simulink model "simSmc"  (R2015b)
settings: Solver=VariableStepAuto  StartTime=0.0  StopTime=10  RelTol=1e-3
InitFcn:
  | run smc.m
values from neighbouring files (symbols this model uses):
  A = [ 0 1; 0 -b]    [constants.m]    (also in smc.m = 500)
  a = g/l    (= 32.1639344262)    [constants.m]    (also in lyapRedesign.m = -10.9; smc.m = -32.1639344262)
  a1 = 12    [smc.m]
  a_hat = g/l_hat    (= -9.81)    [lyapRedesign.m]
  alpha = max(alpha_p)    [smc.m]
  b_hat = k_hat/m_hat    (= 0.151515151515)    [lyapRedesign.m]    (also in smc.m = mean(b_p))
  beta0 = ceil(Rho) - Rho    [smc.m]
  beta_wo_dis = beta_0_wo_dis + Rho_wo_dis    [smc.m]
  c_hat = 1/(m_hat*l_hat^2)    (= 1.51515151515)    [lyapRedesign.m]    (also in smc.m = mean(c_p))
  dt = 1/200    (= 0.005)    [smc.m]
  e = (xLimit/b)^2    (= 0.000625)    [lyapRedesign.m]    (also in smc.m = (x2_bound)/norm(1-1/theta))
  g = 9.81    [constants.m]    (also in lyapRedesign.m = -9.81; smc.m = -9.81)
  k1 = 40    [lyapRedesign.m]
  k2 = 40 - b_hat    (= 39.8484848485)    [lyapRedesign.m]
  Kf = min(Kf_p)    [smc.m]
  Km = 0.0934    [smc.m]
  l = 0.305    [constants.m]    (also in lyapRedesign.m = 0.9; smc.m)
  m = 0.1    [constants.m]    (also in lyapRedesign.m = 1.5; smc.m = min(m_p))
  rho1 = 1/c_hat * (abs((a_hat*c - a*c_hat)/c_hat) + abs((c*b_hat - c_hat*b)/c_hat) + k0*sqrt(5))    [lyapRedesign.m]    (also in smc.m = [abs( (1/c_hat - 1/max(c_p))*a ) abs( (a1-min(b_p))/min(c_p))
  rho2 = m_hat    (= 0.66)    [lyapRedesign.m]    (also in smc.m = (Km*A*(5/2000)/(min(m_p)*l))/min(c_p))
undefined symbols (not defined in the file or in its folder): DiscIntNeverNeededParam
settings Model: Creator=jn  LastModifiedBy=jn

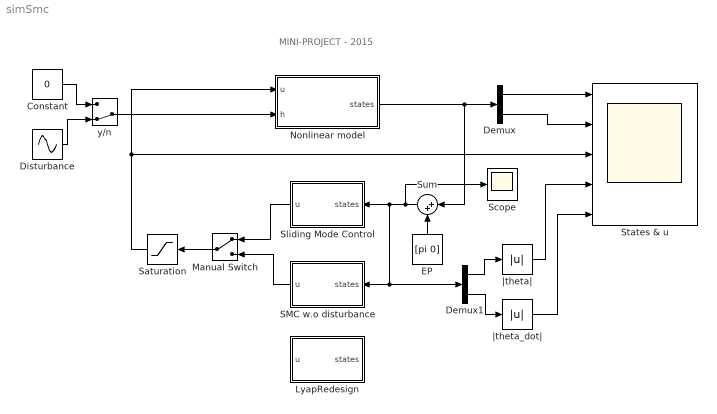
== system simSmc ==
  note: MINI-PROJECT - 2015
  Constant : Constant  Value=0
  Demux : Demux  Outputs=2
  Demux1 : Demux  Outputs=2
  Disturbance : Sin  Amplitude=Km*A*5/2000  SampleTime=0
  EP : Constant  Value=[pi 0]
  LyapRedesign : Subsystem
  Manual Switch : ManualSwitch
  Nonlinear model : Subsystem
  SMC w.o disturbance : Subsystem
  Saturation : Saturate  UpperLimit=2000  LowerLimit=-2000
  Scope : Scope
  Sliding Mode Control : Subsystem
  States & u : Scope  NumInputPorts=5
  Sum : Sum  Inputs=|++
  y/n : ManualSwitch  CurrentSetting=0
  |theta_dot| : Abs
  |theta| : Abs
  wires:
  Nonlinear model/1(states) -> Demux/1, Sum/1
  Demux/1 -> States & u/1
  Demux/2 -> States & u/2
  EP/1 -> Sum/2
  Sum/1 -> Scope/1, Sliding Mode Control/1(states), SMC w.o disturbance/1(states), Demux1/1
  Saturation/1 -> States & u/3, Nonlinear model/1(u)
  Demux1/1 -> |theta|/1
  Demux1/2 -> |theta_dot|/1
  |theta|/1 -> States & u/4
  |theta_dot|/1 -> States & u/5
  SMC w.o disturbance/1(u) -> Manual Switch/2
  Sliding Mode Control/1(u) -> Manual Switch/1
  Manual Switch/1 -> Saturation/1
  Disturbance/1 -> y/n/2
  Constant/1 -> y/n/1
  y/n/1 -> Nonlinear model/2(h)

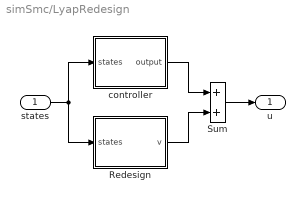
== system simSmc/LyapRedesign ==
  states : Inport
  Redesign : Subsystem
  Sum : Sum
  controller : Subsystem
  u : Outport
  wires:
  states/1 -> controller/1(states), Redesign/1(states)
  Redesign/1(v) -> Sum/2
  controller/1(output) -> Sum/1
  Sum/1 -> u/1

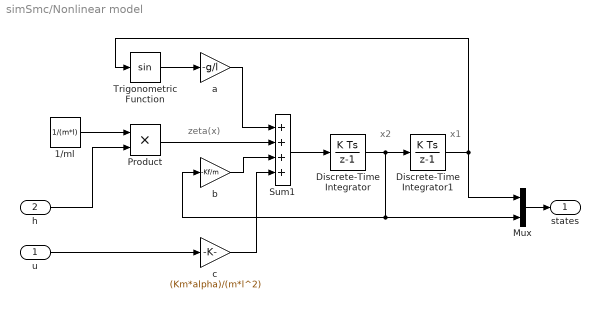
== system simSmc/Nonlinear model ==
  note: zeta(x)
  note: x1
  note: x2
  u : Inport
  h : Inport  Port=2
  1/ml : Constant  Value=1/(m*l)
  Discrete-Time Integrator : DiscreteIntegrator  InitialConditionSetting=State (most efficient)  SampleTime=dt  ICPrevOutput=DiscIntNeverNeededParam  ICPrevScaledInput=DiscIntNeverNeededParam
  Discrete-Time Integrator1 : DiscreteIntegrator  InitialConditionSetting=State (most efficient)  SampleTime=dt  ICPrevOutput=DiscIntNeverNeededParam  ICPrevScaledInput=DiscIntNeverNeededParam
  Mux : Mux  Inputs=2
  Product : Product
  Sum1 : Sum  Inputs=++++
  Trigonometric Function : Trigonometry
  a : Gain  Gain=-g/l
  b : Gain  Gain=-Kf/m
  c : Gain  Gain=(Km*alpha)/(m*l^2)
  states : Outport
  wires:
  u/1 -> c/1
  Trigonometric Function/1 -> a/1
  a/1 -> Sum1/1
  Sum1/1 -> Discrete-Time Integrator/1
  Discrete-Time Integrator/1 -> Discrete-Time Integrator1/1, Mux/2, b/1
  Discrete-Time Integrator1/1 -> Trigonometric Function/1, Mux/1
  Mux/1 -> states/1
  h/1 -> Product/2
  Product/1 -> Sum1/2
  b/1 -> Sum1/3
  c/1 -> Sum1/4
  1/ml/1 -> Product/1

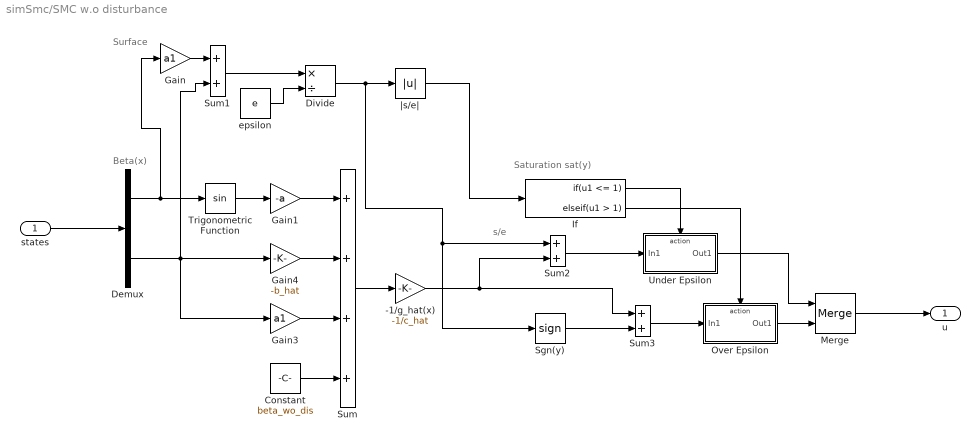
== system simSmc/SMC w.o disturbance ==
  note: Beta(x)
  note: s/e
  note: Saturation sat(y)
  note: Surface
  states : Inport
  -1/g_hat(x) : Gain  Gain=-1/c_hat
  Constant : Constant  Value=beta_wo_dis
  Demux : Demux  Outputs=2
  Divide : Product  Inputs=*/
  Gain : Gain  Gain=a1
  Gain1 : Gain  Gain=-a
  Gain3 : Gain  Gain=a1
  Gain4 : Gain  Gain=-b_hat
  If : If  IfExpression=u1 <= 1  ElseIfExpressions=u1 > 1  ShowElse=off  ZeroCross=off
  Merge : Merge
  Over Epsilon : Subsystem  TreatAsAtomicUnit=on
  Sgn(y) : Signum
  Sum : Sum  Inputs=++++
  Sum1 : Sum
  Sum2 : Sum
  Sum3 : Sum
  Trigonometric Function : Trigonometry
  Under Epsilon : Subsystem  TreatAsAtomicUnit=on
  epsilon : Constant  Value=e
  |s/e| : Abs
  u : Outport
  wires:
  states/1 -> Demux/1
  Demux/1 -> Trigonometric Function/1, Gain/1
  Demux/2 -> Gain4/1, Gain3/1, Sum1/2
  Sum1/1 -> Divide/1
  epsilon/1 -> Divide/2
  |s/e|/1 -> If/1
  If/1 -> Under Epsilon/Action
  Under Epsilon/1(Out1) -> Merge/1
  If/2 -> Over Epsilon/Action
  Over Epsilon/1(Out1) -> Merge/2
  Gain/1 -> Sum1/1
  Trigonometric Function/1 -> Gain1/1
  Gain1/1 -> Sum/1
  Gain3/1 -> Sum/3
  Gain4/1 -> Sum/2
  Sum/1 -> -1/g_hat(x)/1
  Sgn(y)/1 -> Sum3/2
  Divide/1 -> Sum2/1, Sgn(y)/1, |s/e|/1
  Sum2/1 -> Under Epsilon/1(In1)
  Sum3/1 -> Over Epsilon/1(In1)
  Merge/1 -> u/1
  Constant/1 -> Sum/4
  -1/g_hat(x)/1 -> Sum3/1, Sum2/2

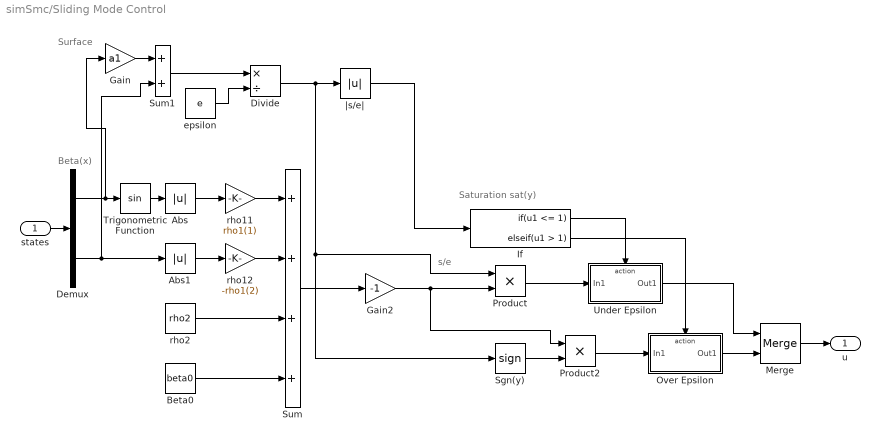
== system simSmc/Sliding Mode Control ==
  note: Beta(x)
  note: s/e
  note: Saturation sat(y)
  note: Surface
  states : Inport
  Abs : Abs
  Abs1 : Abs
  Beta0 : Constant  Value=beta0
  Demux : Demux  Outputs=2
  Divide : Product  Inputs=*/
  Gain : Gain  Gain=a1
  Gain2 : Gain  Gain=-1
  If : If  IfExpression=u1 <= 1  ElseIfExpressions=u1 > 1  ShowElse=off  ZeroCross=off
  Merge : Merge
  Over Epsilon : Subsystem  TreatAsAtomicUnit=on
  Product : Product
  Product2 : Product
  Sgn(y) : Signum
  Sum : Sum  Inputs=++++
  Sum1 : Sum
  Trigonometric Function : Trigonometry
  Under Epsilon : Subsystem  TreatAsAtomicUnit=on
  epsilon : Constant  Value=e
  rho11 : Gain  Gain=rho1(1)
  rho12 : Gain  Gain=-rho1(2)
  rho2 : Constant  Value=rho2
  |s/e| : Abs
  u : Outport
  wires:
  states/1 -> Demux/1
  Sum/1 -> Gain2/1
  Sum1/1 -> Divide/1
  epsilon/1 -> Divide/2
  Gain2/1 -> Product/2, Product2/1
  |s/e|/1 -> If/1
  If/1 -> Under Epsilon/Action
  Merge/1 -> u/1
  Under Epsilon/1(Out1) -> Merge/1
  Product/1 -> Under Epsilon/1(In1)
  Sgn(y)/1 -> Product2/2
  If/2 -> Over Epsilon/Action
  Product2/1 -> Over Epsilon/1(In1)
  Over Epsilon/1(Out1) -> Merge/2
  Gain/1 -> Sum1/1
  rho11/1 -> Sum/1
  Demux/1 -> Trigonometric Function/1, Gain/1
  Demux/2 -> Abs1/1, Sum1/2
  rho12/1 -> Sum/2
  Beta0/1 -> Sum/4
  rho2/1 -> Sum/3
  Abs/1 -> rho11/1
  Abs1/1 -> rho12/1
  Trigonometric Function/1 -> Abs/1
  Divide/1 -> Sgn(y)/1, Product/1, |s/e|/1

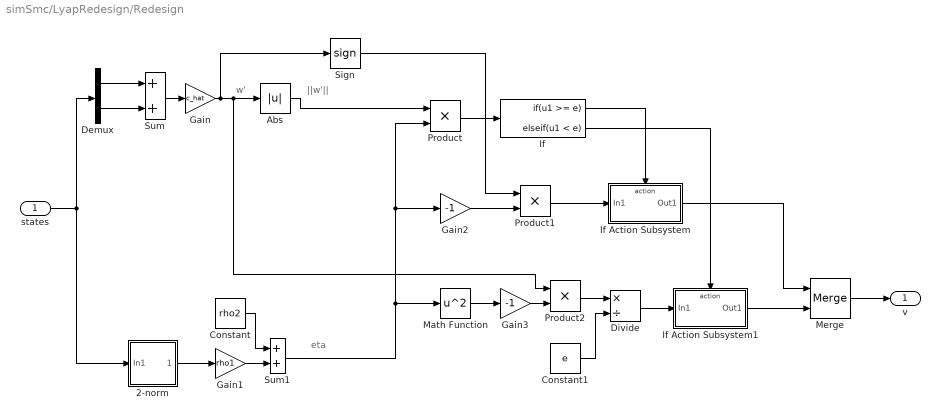
== system simSmc/LyapRedesign/Redesign ==
  note: w'
  note: eta
  note: ||w'||
  states : Inport
  2-norm : Subsystem
  Abs : Abs  ZeroCross=off
  Constant : Constant  Value=rho2
  Constant1 : Constant  Value=e
  Demux : Demux  Outputs=2
  Divide : Product  Inputs=*/
  Gain : Gain  Gain=c_hat
  Gain1 : Gain  Gain=rho1
  Gain2 : Gain  Gain=-1
  Gain3 : Gain  Gain=-1
  If : If  IfExpression=u1 >= e  ElseIfExpressions=u1 < e  ShowElse=off  ZeroCross=off
  If Action Subsystem : Subsystem  TreatAsAtomicUnit=on
  If Action Subsystem1 : Subsystem  TreatAsAtomicUnit=on
  Math Function : Math  Operator=square  SaturateOnIntegerOverflow=on
  Merge : Merge
  Product : Product
  Product1 : Product
  Product2 : Product
  Sign : Signum  ZeroCross=off
  Sum : Sum
  Sum1 : Sum
  v : Outport
  wires:
  states/1 -> 2-norm/1(In1), Demux/1
  Demux/2 -> Sum/2
  Demux/1 -> Sum/1
  Sum/1 -> Gain/1
  Gain/1 -> Sign/1, Product2/1, Abs/1
  2-norm/1(Out1) -> Gain1/1
  Gain1/1 -> Sum1/2
  Constant/1 -> Sum1/1
  Sum1/1 -> Gain2/1, Product/2, Math Function/1
  Abs/1 -> Product/1
  Product/1 -> If/1
  If/1 -> If Action Subsystem/Action
  Gain2/1 -> Product1/2
  Sign/1 -> Product1/1
  Product1/1 -> If Action Subsystem/1(In1)
  Merge/1 -> v/1
  If Action Subsystem/1(Out1) -> Merge/1
  Math Function/1 -> Gain3/1
  Gain3/1 -> Product2/2
  Constant1/1 -> Divide/2
  Product2/1 -> Divide/1
  Divide/1 -> If Action Subsystem1/1(In1)
  If Action Subsystem1/1(Out1) -> Merge/2
  If/2 -> If Action Subsystem1/Action

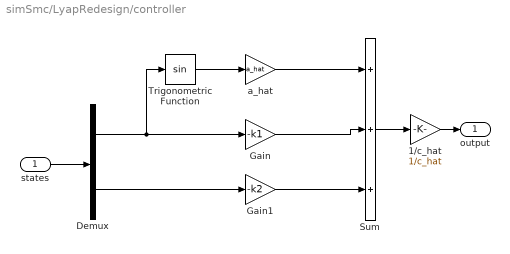
== system simSmc/LyapRedesign/controller ==
  states : Inport
  1/c_hat : Gain  Gain=1/c_hat
  Demux : Demux  Outputs=2
  Gain : Gain  Gain=-k1
  Gain1 : Gain  Gain=-k2
  Sum : Sum  Inputs=+++
  Trigonometric Function : Trigonometry
  a_hat : Gain  Gain=a_hat
  output : Outport
  wires:
  states/1 -> Demux/1
  Demux/1 -> Trigonometric Function/1, Gain/1
  Demux/2 -> Gain1/1
  Trigonometric Function/1 -> a_hat/1
  a_hat/1 -> Sum/1
  Gain/1 -> Sum/2
  Gain1/1 -> Sum/3
  1/c_hat/1 -> output/1
  Sum/1 -> 1/c_hat/1

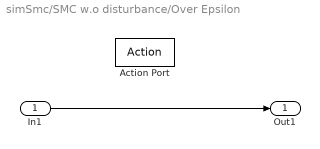
== system simSmc/SMC w.o disturbance/Over Epsilon ==
  In1 : Inport
  Action Port : ActionPort  ActionType=elseif
  Out1 : Outport
  wires:
  In1/1 -> Out1/1

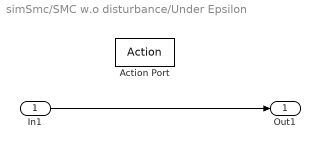
== system simSmc/SMC w.o disturbance/Under Epsilon ==
  In1 : Inport
  Action Port : ActionPort  ActionType=then
  Out1 : Outport
  wires:
  In1/1 -> Out1/1

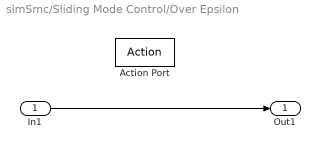
== system simSmc/Sliding Mode Control/Over Epsilon ==
  In1 : Inport
  Action Port : ActionPort  ActionType=elseif
  Out1 : Outport
  wires:
  In1/1 -> Out1/1

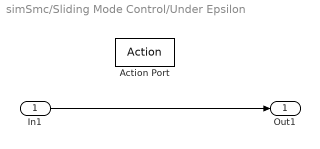
== system simSmc/Sliding Mode Control/Under Epsilon ==
  In1 : Inport
  Action Port : ActionPort  ActionType=then
  Out1 : Outport
  wires:
  In1/1 -> Out1/1

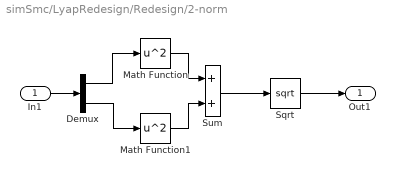
== system simSmc/LyapRedesign/Redesign/2-norm ==
  In1 : Inport
  Demux : Demux  Outputs=2
  Math Function : Math  Operator=square  SaturateOnIntegerOverflow=on
  Math Function1 : Math  Operator=square  SaturateOnIntegerOverflow=on
  Sqrt : Sqrt  SaturateOnIntegerOverflow=on
  Sum : Sum
  Out1 : Outport
  wires:
  In1/1 -> Demux/1
  Demux/1 -> Math Function/1
  Demux/2 -> Math Function1/1
  Math Function1/1 -> Sum/2
  Math Function/1 -> Sum/1
  Sum/1 -> Sqrt/1
  Sqrt/1 -> Out1/1

== system simSmc/LyapRedesign/Redesign/If Action Subsystem ==
  In1 : Inport
  Action Port : ActionPort
  Out1 : Outport
  wires:
  In1/1 -> Out1/1

== system simSmc/LyapRedesign/Redesign/If Action Subsystem1 ==
  In1 : Inport
  Action Port : ActionPort
  Out1 : Outport
  wires:
  In1/1 -> Out1/1
